simulink model "final"  (R2023a)
settings: Solver=VariableStepAuto  StartTime=0.0  StopTime=10.0  RelTol=1e-3
settings Model: Creator=user  LastModifiedBy=diontep

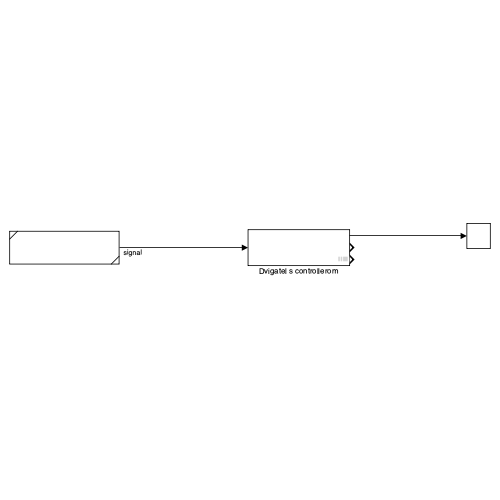
[thumbnail: Simulink's stored preview of the top-level diagram]
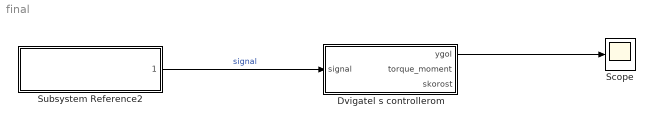
== system final ==
  Dvigatel s controllerom : Subsystem
  Scope : Scope
  Subsystem Reference2 : Subsystem  ReferencedSubsystem=tester  test=3
  wires:
  Subsystem Reference2/1 -> Dvigatel s controllerom/1(signal)  "signal"
  Dvigatel s controllerom/1(ygol) -> Scope/1

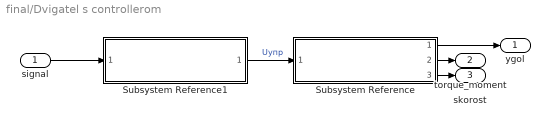
== system final/Dvigatel s controllerom ==
  signal : Inport
  Subsystem Reference : Subsystem  ReferencedSubsystem=dvigatel  J=7e-6  Cm=1.3  Cw=3.15  L=0.0015  R=8  Lob=0.013  b=0.001
  Subsystem Reference1 : Subsystem  ReferencedSubsystem=connector  k1=5  k2=8  k3=12
  ygol : Outport
  torque_moment : Outport  Port=2
  skorost : Outport  Port=3
  wires:
  signal/1 -> Subsystem Reference1/1
  Subsystem Reference/3 -> skorost/1
  Subsystem Reference/2 -> torque_moment/1
  Subsystem Reference/1 -> ygol/1
  Subsystem Reference1/1 -> Subsystem Reference/1  "Uупр"
